simulink model "Simulink_model"  (R2025b)
settings: Solver=FixedStepAuto  StartTime=0.0  StopTime=20  FixedStep=1e-3  RelTol=1e-3
values from neighbouring files (symbols this model uses):
  b = 0.05    [Data.m]
  g = 9.81    [Data.m]
  l = 0.25    [Data.m]
  m = 1    [Data.m]
  theta0 = deg2rad(theta0_deg)    [Data.m]
  theta0dot = deg2rad(theta0dot_deg)    [Data.m]
settings Model: Creator=Enrico 2  LastModifiedBy=Enrico 2

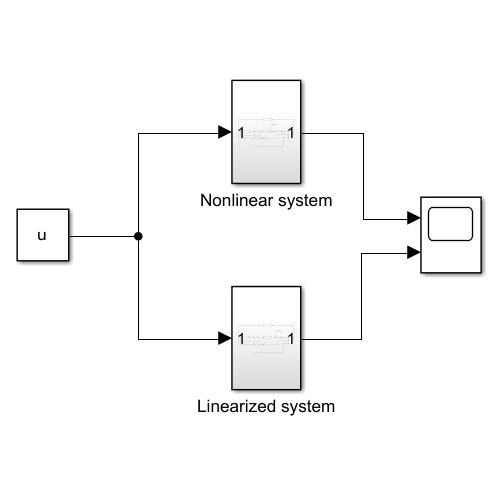
[thumbnail: Simulink's stored preview of the top-level diagram]
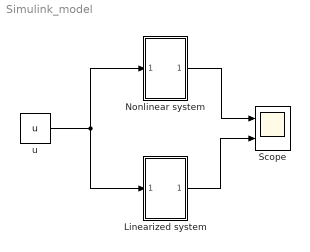
== system Simulink_model ==
  Linearized system : Subsystem
  Nonlinear system : Subsystem
  Scope : Scope  NumInputPorts=2
      settings: ActiveDisplayYMinimum=-0.18240996565774259  ActiveDisplayYMaximum=0.2141932464057858
  u : Constant  Value=u
  wires:
  u/1 -> Linearized system/1(In1), Nonlinear system/1(In1)
  Nonlinear system/1(Out1) -> Scope/1
  Linearized system/1(Out1) -> Scope/2

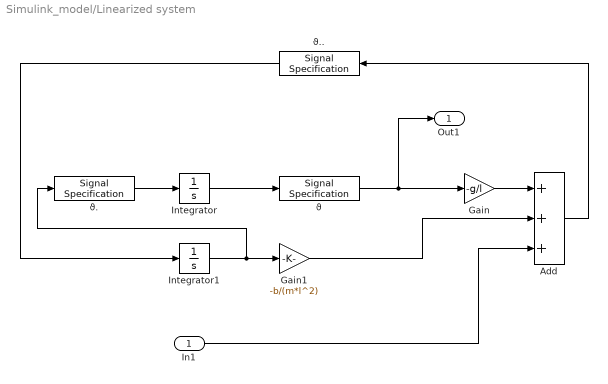
== system Simulink_model/Linearized system ==
  In1 : Inport
  Add : Sum  Inputs=+++
  Gain : Gain  Gain=-g/l
  Gain1 : Gain  Gain=-b/(m*l^2)
  Integrator : Integrator  InitialCondition=theta0
  Integrator1 : Integrator  InitialCondition=theta0dot
  ϑ : SignalSpecification  Unit=rad
  ϑ. : SignalSpecification  Unit=rad/sec
  ϑ.. : SignalSpecification  Unit=rad/sec^2
  Out1 : Outport
  wires:
  Integrator1/1 -> ϑ./1, Gain1/1
  Integrator/1 -> ϑ/1
  ϑ/1 -> Gain/1, Out1/1
  In1/1 -> Add/3
  Gain1/1 -> Add/2
  ϑ../1 -> Integrator1/1
  Gain/1 -> Add/1
  Add/1 -> ϑ../1
  ϑ./1 -> Integrator/1

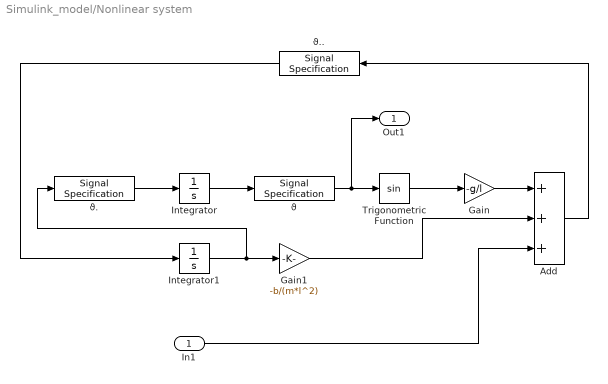
== system Simulink_model/Nonlinear system ==
  In1 : Inport
  Add : Sum  Inputs=+++
  Gain : Gain  Gain=-g/l
  Gain1 : Gain  Gain=-b/(m*l^2)
  Integrator : Integrator  InitialCondition=theta0
  Integrator1 : Integrator  InitialCondition=theta0dot
  Trigonometric Function : Trigonometry
  ϑ : SignalSpecification  Unit=rad
  ϑ. : SignalSpecification  Unit=rad/sec
  ϑ.. : SignalSpecification  Unit=rad/sec^2
  Out1 : Outport
  wires:
  Integrator1/1 -> ϑ./1, Gain1/1
  Integrator/1 -> ϑ/1
  ϑ/1 -> Out1/1, Trigonometric Function/1
  In1/1 -> Add/3
  Gain1/1 -> Add/2
  ϑ../1 -> Integrator1/1
  Gain/1 -> Add/1
  Add/1 -> ϑ../1
  ϑ./1 -> Integrator/1
  Trigonometric Function/1 -> Gain/1
